simulink model "SSB_AWGN"  (R2023a)
settings: Solver=VariableStepAuto  StartTime=0.0  StopTime=1  RelTol=1e-3
libraries: dspfdesign x2, commchan3 x1
settings Model: Creator=Pedro  LastModifiedBy=Pedro

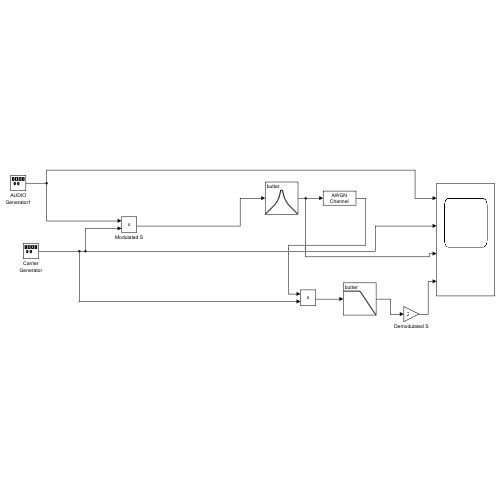
[thumbnail: Simulink's stored preview of the top-level diagram]
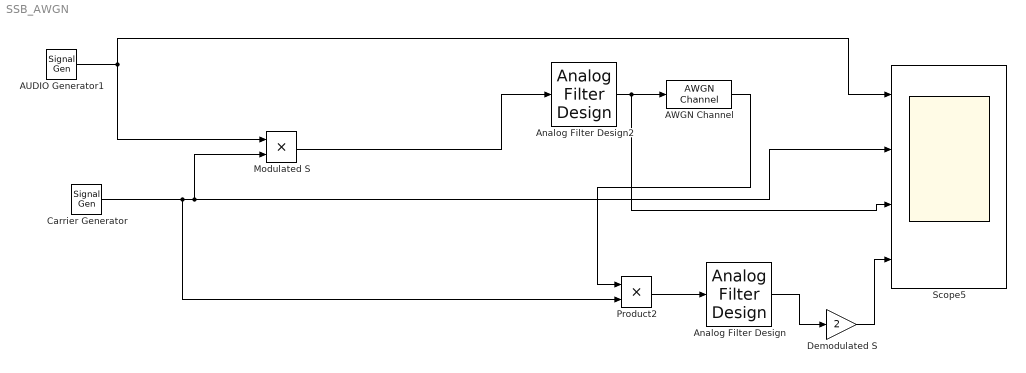
== system SSB_AWGN ==
  AUDIO Generator1 : SignalGenerator  Amplitude=1.5  Frequency=20  VectorParams1D=off
  AWGN Channel : commchan3/AWGN Channel  LegacyMode=off  NoiseMethod="Signal to noise ratio  (SNR)"  noiseMode="Signal to noise ratio  (SNR)"  EbNo=10  EsNo=10  SNR=23  BitsPerSymbol=1  SignalPower=1  SamplesPerSymbol=1  SymbolPeriod=1  VarianceSource=Parameter  Variance=1  RandomStream=Global stream  Seed=67  SimulateUsing=Code generation
  Analog Filter Design : dspfdesign/Analog Filter Design  method=Butterworth  filttype=Lowpass  N=8  Wlo=2*pi*90  Whi=2*pi*1000  Rp=2  Rs=40
  Analog Filter Design2 : dspfdesign/Analog Filter Design  method=Butterworth  filttype=Bandpass  N=8  Wlo=2*pi*80  Whi=2*pi*100  Rp=2  Rs=40
  Carrier Generator : SignalGenerator  Frequency=110
  Demodulated S : Gain  Gain=2
  Modulated S : Product
  Product2 : Product
  Scope5 : Scope  NumInputPorts=4
  wires:
  Demodulated S/1 -> Scope5/4
  Carrier Generator/1 -> Scope5/2, Modulated S/2, Product2/2
  Modulated S/1 -> Analog Filter Design2/1
  Analog Filter Design/1 -> Demodulated S/1
  Product2/1 -> Analog Filter Design/1
  AUDIO Generator1/1 -> Scope5/1, Modulated S/1
  Analog Filter Design2/1 -> Scope5/3, AWGN Channel/1
  AWGN Channel/1 -> Product2/1
